simulink model "Onduleur"  (R2019b)
settings: Solver=VariableStepAuto  StartTime=0.0  StopTime=0.04  RelTol=1e-3
libraries: simulink x1
settings Model: Creator=x1 yoga  LastModifiedBy=x1 yoga

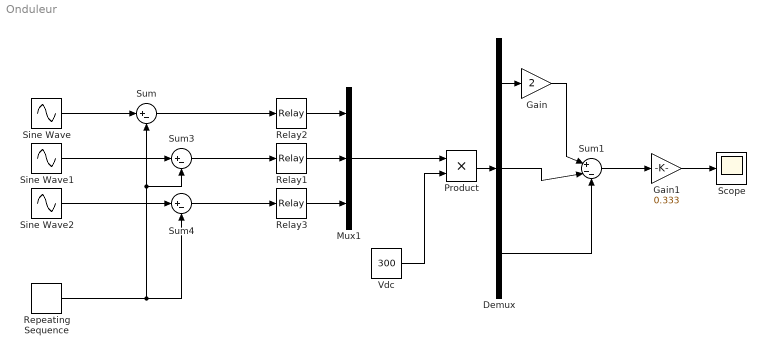
== system Onduleur ==
  Demux : Demux  Outputs=3
  Gain : Gain  Gain=2
  Gain1 : Gain  Gain=0.333
  Mux1 : Mux  Inputs=3
  Product : Product
  Relay1 : Relay  OnSwitchValue=0.1  OffSwitchValue=-0.1  OffOutputValue=-1
  Relay2 : Relay  OnSwitchValue=0.1  OffSwitchValue=-0.1  OffOutputValue=-1
  Relay3 : Relay  OnSwitchValue=0.1  OffSwitchValue=-0.1  OffOutputValue=-1
  Repeating Sequence : simulink/Sources/Repeating Sequence  rep_seq_t=[0 0.00025 0.0005]  rep_seq_y=[0 1 0]
  Scope : Scope
  Sine Wave : Sin  Amplitude=100  Frequency=2*pi*50  SampleTime=0
  Sine Wave1 : Sin  Amplitude=100  Frequency=2*pi*50  Phase=-2*pi/3  SampleTime=0
  Sine Wave2 : Sin  Amplitude=100  Frequency=2*pi*50  Phase=2*pi/3  SampleTime=0
  Sum : Sum  Inputs=|+-
  Sum1 : Sum  Inputs=|+--
  Sum3 : Sum  Inputs=|+-
  Sum4 : Sum  Inputs=|+-
  "Vdc " : Constant  Value=300
  wires:
  Sine Wave/1 -> Sum/1
  Sine Wave1/1 -> Sum3/1
  Sine Wave2/1 -> Sum4/1
  Repeating Sequence/1 -> Sum3/2, Sum/2, Sum4/2
  Sum/1 -> Relay2/1
  Sum3/1 -> Relay1/1
  Sum4/1 -> Relay3/1
  "Vdc "/1 -> Product/2
  Product/1 -> Demux/1
  Relay2/1 -> Mux1/1
  Relay1/1 -> Mux1/2
  Relay3/1 -> Mux1/3
  Mux1/1 -> Product/1
  Demux/1 -> Gain/1
  Gain/1 -> Sum1/1
  Demux/2 -> Sum1/2
  Demux/3 -> Sum1/3
  Sum1/1 -> Gain1/1
  Gain1/1 -> Scope/1
